simulink model "interface"  (R2018b)
settings: Solver=FixedStepDiscrete  StartTime=0.0  StopTime=10.0  RelTol=1e-3
settings Model: Creator=matlab  LastModifiedBy=matlab

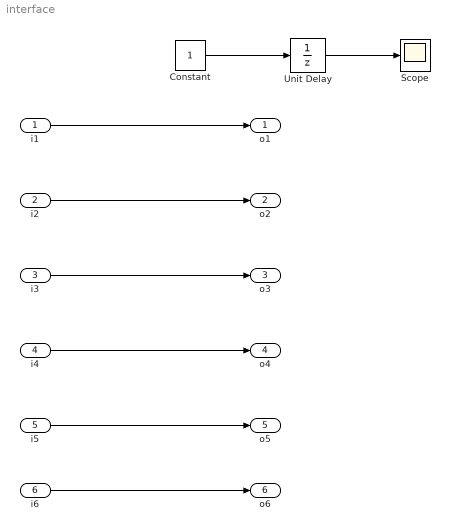
== system interface ==
  i1 : Inport  OutDataTypeStr=Enum: BoolSimulinkIntEnumType
  i2 : Inport  Port=2  OutDataTypeStr=Enum: BoolUInt8Enum
  i3 : Inport  Port=3  OutDataTypeStr=Enum: BoolUInt16Enum
  i4 : Inport  Port=4  OutDataTypeStr=Enum: BoolInt8Enum
  i5 : Inport  Port=5  OutDataTypeStr=Enum: BoolInt16Enum
  i6 : Inport  Port=6  OutDataTypeStr=Enum: BoolInt32Enum
  Constant : Constant
  Scope : Scope
  Unit Delay : UnitDelay  SampleTime=-1
  o1 : Outport  OutDataTypeStr=Enum: BoolSimulinkIntEnumType
  o2 : Outport  Port=2  OutDataTypeStr=Enum: BoolUInt8Enum
  o3 : Outport  Port=3  OutDataTypeStr=Enum: BoolUInt16Enum
  o4 : Outport  Port=4  OutDataTypeStr=Enum: BoolInt8Enum
  o5 : Outport  Port=5  OutDataTypeStr=Enum: BoolInt16Enum
  o6 : Outport  Port=6  OutDataTypeStr=Enum: BoolInt32Enum
  wires:
  i3/1 -> o3/1
  i2/1 -> o2/1
  i5/1 -> o5/1
  i6/1 -> o6/1
  i4/1 -> o4/1
  i1/1 -> o1/1
  Unit Delay/1 -> Scope/1
  Constant/1 -> Unit Delay/1
